simulink model "Two_Channel_PP_Teleoperation_kalman"  (R2022b)
settings: Solver=VariableStepAuto  StartTime=0.0  StopTime=10  RelTol=1e-9
values from neighbouring files (symbols this model uses):
  Amp = 15    [parameters.m]    (also in parameters_kalman.m)
  Be = 100    [parameters.m]    (also in parameters_kalman.m)
  Bh = 1    [parameters.m]    (also in parameters_kalman.m)
  Bm = 20*0.8    (= 16)    [parameters.m]    (also in parameters_kalman.m = 80)
  Bs = 4*Bm    (= 64)    [parameters.m]    (also in parameters_kalman.m = 300)
  delay = 10    [parameters.m]    (also in parameters_kalman.m)
  Dh = 20*0.8    (= 16)    [parameters.m]    (also in parameters_kalman.m)
  Dm = 1.3    [parameters.m]    (also in parameters_kalman.m)
  Ds = 1.2    [parameters.m]    (also in parameters_kalman.m)
  Fc = 1    [parameters.m]    (also in parameters_kalman.m)
  Flp = 5    [parameters.m]    (also in parameters_kalman.m)
  Jh = 1    [parameters.m]    (also in parameters_kalman.m)
  Ke = 200    [parameters.m]    (also in parameters_kalman.m)
  Km = 10*1    (= 10)    [parameters.m]    (also in parameters_kalman.m = 30)
  Ks = 4*Km    (= 40)    [parameters.m]    (also in parameters_kalman.m = 240)
  lambda = 150    [parameters_kalman.m]
  Mm = 0.5    [parameters.m]    (also in parameters_kalman.m)
  Ms = 2    [parameters.m]    (also in parameters_kalman.m)
  Ph = 10*1    (= 10)    [parameters.m]    (also in parameters_kalman.m)
  Ts = 0.001    [parameters.m]    (also in parameters_kalman.m)
  variance = 0.000001    (= 1e-06)    [parameters_kalman.m]
  xe = 1000    [parameters.m]    (also in parameters_kalman.m = 30)
undefined symbols (not defined in the file or in its folder): DiscIntNeverNeededParam
libraries: simulink x2
settings Model: Creator=uzair  LastModifiedBy=uzair

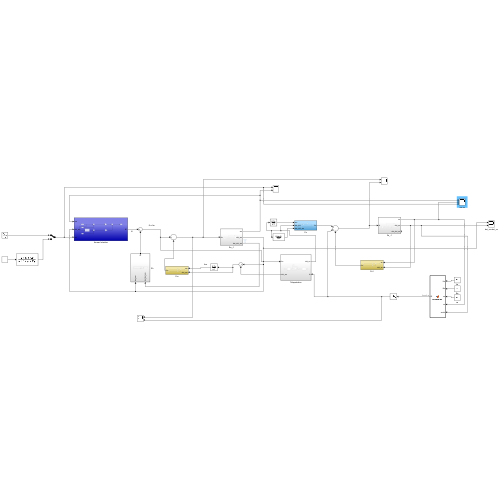
[thumbnail: Simulink's stored preview of the top-level diagram]
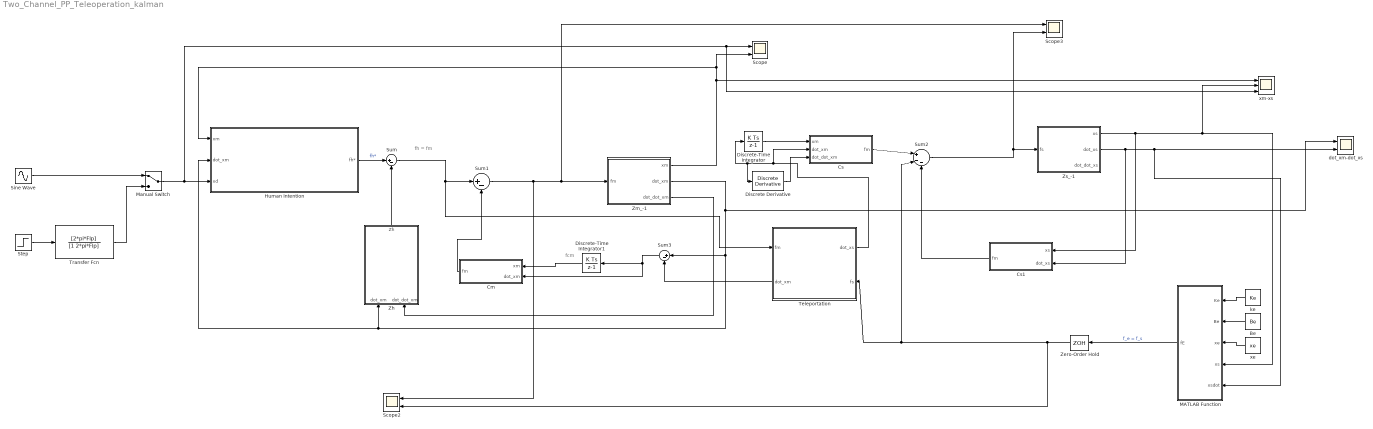
== system Two_Channel_PP_Teleoperation_kalman ==
  note: fcm
  note: fh = fm
  Be : Constant  Value=Be
  Cm : Subsystem
  Cs : Subsystem
  Cs1 : Subsystem
  Discrete Derivative : simulink/Discrete/Discrete Derivative  gainval=1.0  ICPrevScaledInput=0.0  OutMin=[]  OutMax=[]  OutDataType=fixdt(1, 16)  OutScaling=2^-10  DoSatur=off
  Discrete-Time Integrator : DiscreteIntegrator  SampleTime=Ts  ICPrevOutput=DiscIntNeverNeededParam  ICPrevScaledInput=DiscIntNeverNeededParam
  Discrete-Time Integrator1 : DiscreteIntegrator  SampleTime=Ts  ICPrevOutput=DiscIntNeverNeededParam  ICPrevScaledInput=DiscIntNeverNeededParam
  Human Intention : Subsystem
  MATLAB Function : MATLAB Function  TreatAsAtomicUnit=on
  Manual Switch : ManualSwitch
  Scope : Scope  NumInputPorts=2
  Scope2 : Scope  NumInputPorts=2
  Scope3 : Scope  NumInputPorts=2
  Sine Wave : Sin  Amplitude=Amp  Frequency=2*pi*Fc  SampleTime=0
  Step : Step  Time=0.5  After=Amp  SampleTime=0
  Sum : Sum  Inputs=|+-
  Sum1 : Sum  Inputs=|+-
  Sum2 : Sum  Inputs=|+--
  Sum3 : Sum  Inputs=|+-
  Teleportation : Subsystem
      settings: PortSchema="{\"entries\":[{\"content\":{\"sides\":[{\"content\":{\"connectorIds\":[\"In1\",\"Out2\"]},\"type\":\"ConnectorPlacement.EquallySpacedRectSide\",\"uuid\":\"b5f7abc7-c75d-4363-a17a-8f86c90608cd\"},{\"content\":{\"connectorIds\":[\"Out1\",\"In2\"],\"side\":\"RIGHT\"},\"type\":\"ConnectorPlacement.EquallySpacedRectSide\",\"uuid\":\"2ed87bee-e320-4c73-a1d3-1960a55b558d\"},{\"content\":{\"connectorIds\":[],\"side\":\"TOP\"},\"type\":\"ConnectorPlacement.EquallySpacedRectSide\",\"uuid\":\"65d6df07-20ed-40e6-978a-52c206d58fbe\"}]},\"type\":\"ConnectorPlacement.EquallySpacedConnector\",\"uuid\":\"b3d72d1f-cf16-401b-a692-293857f5cfdb\"}],\"packageUris\":[\"http://schema.mathworks.com/mf0/Connector/R2020b\"],\"version\":\"1.0\"}"
  Transfer Fcn : TransferFcn  Numerator=[2*pi*Flp]  Denominator=[1 2*pi*Flp]
  Zero-Order Hold : ZeroOrderHold  SampleTime=Ts
  Zh : Subsystem
  Zm_-1 : Subsystem
  Zs_-1 : Subsystem
  dot_xm-dot_xs : Scope  NumInputPorts=2
  ke : Constant  Value=Ke
  xe : Constant  Value=xe
  xm-xs : Scope  NumInputPorts=3
  wires:
  Sine Wave/1 -> Manual Switch/1
  Step/1 -> Transfer Fcn/1
  Transfer Fcn/1 -> Manual Switch/2
  Manual Switch/1 -> xm-xs/3, Scope/1, Human Intention/3(xd)
  Human Intention/1(fh*) -> Sum/1  "fh*"
  Zh/1(Zh) -> Sum/2
  Sum/1 -> Sum1/1, Teleportation/1(fm)
  Sum1/1 -> Scope2/1, Scope3/1, Zm_-1/1(fm)
  Zm_-1/3(dot_dot_xm) -> Zh/2(dot_dot_xm)
  Zm_-1/2(dot_xm) -> dot_xm-dot_xs/1, Human Intention/2(dot_xm), Zh/1(dot_xm), Sum3/1
  Cm/1(fm) -> Sum1/2
  Teleportation/2(dot_xm) -> Sum3/2
  Sum2/1 -> Scope3/2, Zs_-1/1(fs)
  xe/1 -> MATLAB Function/3(xe)
  Be/1 -> MATLAB Function/2(Be)
  ke/1 -> MATLAB Function/1(Ke)
  MATLAB Function/1(fE) -> Zero-Order Hold/1  "f_e = f_s"
  Zm_-1/1(xm) -> Scope/2, Human Intention/1(xm), xm-xs/1
  Cs/1(fm) -> Sum2/1
  Sum3/1 -> Cm/2(dot_xm), Discrete-Time Integrator1/1
  Discrete-Time Integrator1/1 -> Cm/1(xm)
  Zs_-1/2(dot_xs) -> Cs1/2(dot_xs), dot_xm-dot_xs/2, MATLAB Function/5(xsdot)
  Teleportation/1(dot_xs) -> Cs/2(dot_xm), Discrete Derivative/1, Discrete-Time Integrator/1
  Zs_-1/1(xs) -> Cs1/1(xs), xm-xs/2, MATLAB Function/4(xs)
  Zero-Order Hold/1 -> Teleportation/2(fs), Sum2/2, Scope2/2
  Discrete-Time Integrator/1 -> Cs/1(xm)
  Discrete Derivative/1 -> Cs/3(dot_dot_xm)
  Cs1/1(fm) -> Sum2/3

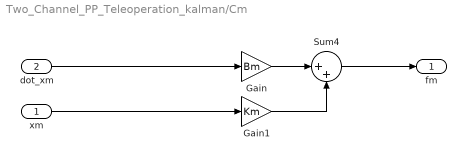
== system Two_Channel_PP_Teleoperation_kalman/Cm ==
  xm : Inport
  dot_xm : Inport  Port=2
  Gain : Gain  Gain=Bm
  Gain1 : Gain  Gain=Km
  Sum4 : Sum  Inputs=|++
  fm : Outport
  wires:
  Sum4/1 -> fm/1
  xm/1 -> Gain1/1
  Gain/1 -> Sum4/1
  Gain1/1 -> Sum4/2
  dot_xm/1 -> Gain/1

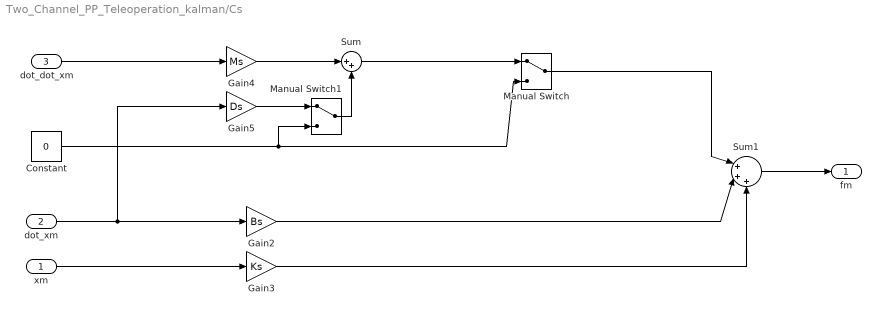
== system Two_Channel_PP_Teleoperation_kalman/Cs ==
  xm : Inport
  dot_xm : Inport  Port=2
  dot_dot_xm : Inport  Port=3
  Constant : Constant  Value=0
  Gain2 : Gain  Gain=Bs
  Gain3 : Gain  Gain=Ks
  Gain4 : Gain  Gain=Ms
  Gain5 : Gain  Gain=Ds
  Manual Switch : ManualSwitch
  Manual Switch1 : ManualSwitch
  Sum : Sum  Inputs=|++
  Sum1 : Sum  Inputs=|+++
  fm : Outport
  wires:
  Manual Switch1/1 -> Sum/2
  dot_xm/1 -> Gain5/1, Gain2/1
  Sum1/1 -> fm/1
  Sum/1 -> Manual Switch/1
  dot_dot_xm/1 -> Gain4/1
  Gain5/1 -> Manual Switch1/1
  Gain4/1 -> Sum/1
  xm/1 -> Gain3/1
  Gain2/1 -> Sum1/2
  Manual Switch/1 -> Sum1/1
  Gain3/1 -> Sum1/3
  Constant/1 -> Manual Switch1/2, Manual Switch/2

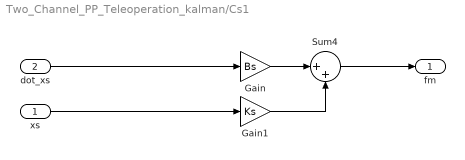
== system Two_Channel_PP_Teleoperation_kalman/Cs1 ==
  xs : Inport
  dot_xs : Inport  Port=2
  Gain : Gain  Gain=Bs
  Gain1 : Gain  Gain=Ks
  Sum4 : Sum  Inputs=|++
  fm : Outport
  wires:
  Sum4/1 -> fm/1
  xs/1 -> Gain1/1
  Gain/1 -> Sum4/1
  Gain1/1 -> Sum4/2
  dot_xs/1 -> Gain/1

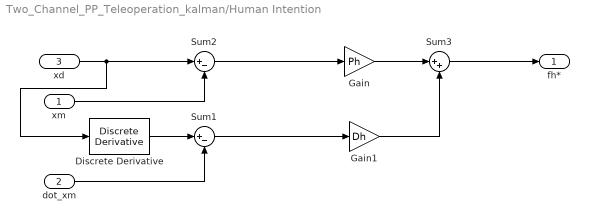
== system Two_Channel_PP_Teleoperation_kalman/Human Intention ==
  xm : Inport
  dot_xm : Inport  Port=2
  xd : Inport  Port=3
  Discrete Derivative : simulink/Discrete/Discrete Derivative  gainval=1.0  ICPrevScaledInput=0.0  OutMin=[]  OutMax=[]  OutDataType=fixdt(1, 16)  OutScaling=2^-10  DoSatur=off
  Gain : Gain  Gain=Ph
  Gain1 : Gain  Gain=Dh
  Sum1 : Sum  Inputs=|+-
  Sum2 : Sum  Inputs=|+-
  Sum3 : Sum  Inputs=|++
  fh* : Outport
  wires:
  xm/1 -> Sum2/2
  dot_xm/1 -> Sum1/2
  Sum2/1 -> Gain/1
  Sum1/1 -> Gain1/1
  Gain1/1 -> Sum3/2
  Gain/1 -> Sum3/1
  Sum3/1 -> fh*/1
  xd/1 -> Discrete Derivative/1, Sum2/1
  Discrete Derivative/1 -> Sum1/1

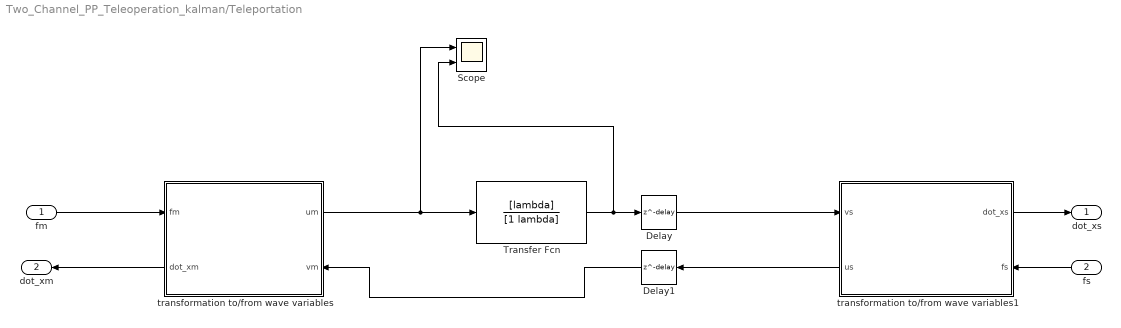
== system Two_Channel_PP_Teleoperation_kalman/Teleportation ==
  fm : Inport
  fs : Inport  Port=2
  Delay : Delay  DelayLength=delay  SampleTime=Ts
  Delay1 : Delay  DelayLength=delay  SampleTime=Ts
  Scope : Scope  NumInputPorts=2
  Transfer Fcn : TransferFcn  Numerator=[lambda]  Denominator=[1 lambda]
  transformation to/from wave variables : Subsystem
      settings: PortSchema="{\"entries\":[{\"content\":{\"sides\":[{\"content\":{\"connectorIds\":[\"In1\",\"Out2\"]},\"type\":\"ConnectorPlacement.EquallySpacedRectSide\",\"uuid\":\"b5f7abc7-c75d-4363-a17a-8f86c90608cd\"},{\"content\":{\"connectorIds\":[\"Out1\",\"In2\"],\"side\":\"RIGHT\"},\"type\":\"ConnectorPlacement.EquallySpacedRectSide\",\"uuid\":\"2ed87bee-e320-4c73-a1d3-1960a55b558d\"},{\"content\":{\"connectorIds\":[],\"side\":\"TOP\"},\"type\":\"ConnectorPlacement.EquallySpacedRectSide\",\"uuid\":\"65d6df07-20ed-40e6-978a-52c206d58fbe\"}]},\"type\":\"ConnectorPlacement.EquallySpacedConnector\",\"uuid\":\"b3d72d1f-cf16-401b-a692-293857f5cfdb\"}],\"packageUris\":[\"http://schema.mathworks.com/mf0/Connector/R2020b\"],\"version\":\"1.0\"}"
  transformation to/from wave variables1 : Subsystem
      settings: PortSchema="{\"entries\":[{\"content\":{\"sides\":[{\"content\":{\"connectorIds\":[\"In1\",\"Out2\"]},\"type\":\"ConnectorPlacement.EquallySpacedRectSide\",\"uuid\":\"b5f7abc7-c75d-4363-a17a-8f86c90608cd\"},{\"content\":{\"connectorIds\":[\"Out1\",\"In2\"],\"side\":\"RIGHT\"},\"type\":\"ConnectorPlacement.EquallySpacedRectSide\",\"uuid\":\"2ed87bee-e320-4c73-a1d3-1960a55b558d\"},{\"content\":{\"connectorIds\":[],\"side\":\"TOP\"},\"type\":\"ConnectorPlacement.EquallySpacedRectSide\",\"uuid\":\"65d6df07-20ed-40e6-978a-52c206d58fbe\"}]},\"type\":\"ConnectorPlacement.EquallySpacedConnector\",\"uuid\":\"b3d72d1f-cf16-401b-a692-293857f5cfdb\"}],\"packageUris\":[\"http://schema.mathworks.com/mf0/Connector/R2020b\"],\"version\":\"1.0\"}"
  dot_xs : Outport
  dot_xm : Outport  Port=2
  wires:
  fm/1 -> transformation to/from wave variables/1(fm)
  transformation to/from wave variables/2(dot_xm) -> dot_xm/1
  fs/1 -> transformation to/from wave variables1/2(fs)
  transformation to/from wave variables1/1(dot_xs) -> dot_xs/1
  transformation to/from wave variables1/2(us) -> Delay1/1
  Delay/1 -> transformation to/from wave variables1/1(vs)
  transformation to/from wave variables/1(um) -> Transfer Fcn/1, Scope/1
  Transfer Fcn/1 -> Scope/2, Delay/1
  Delay1/1 -> transformation to/from wave variables/2(vm)

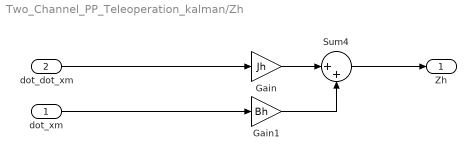
== system Two_Channel_PP_Teleoperation_kalman/Zh ==
  dot_xm : Inport
  dot_dot_xm : Inport  Port=2
  Gain : Gain  Gain=Jh
  Gain1 : Gain  Gain=Bh
  Sum4 : Sum  Inputs=|++
  Zh : Outport
  wires:
  dot_dot_xm/1 -> Gain/1
  Gain1/1 -> Sum4/2
  Gain/1 -> Sum4/1
  Sum4/1 -> Zh/1
  dot_xm/1 -> Gain1/1

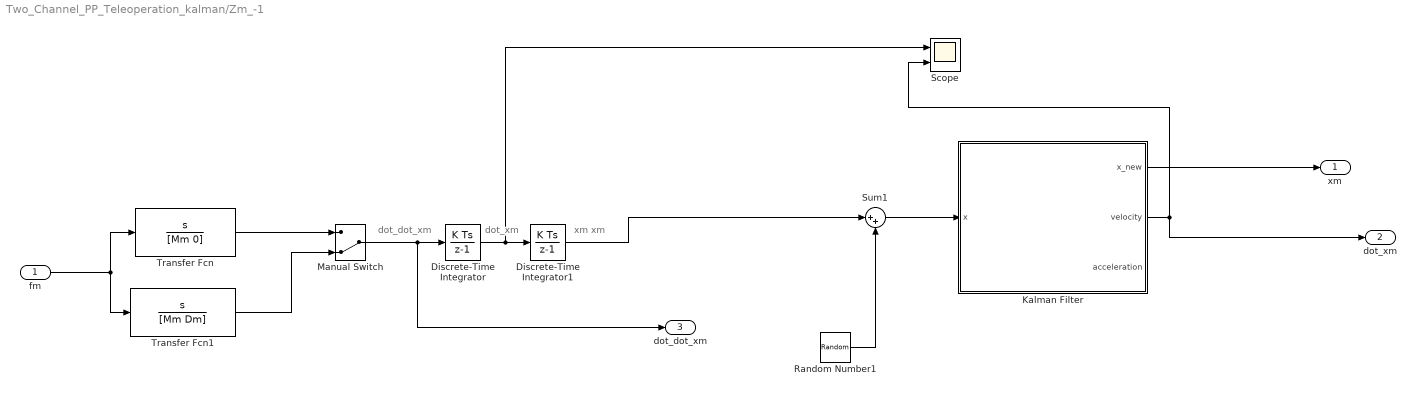
== system Two_Channel_PP_Teleoperation_kalman/Zm_-1 ==
  note: dot_dot_xm
  note: dot_xm
  note: xm
      | xm
  fm : Inport
  Discrete-Time Integrator : DiscreteIntegrator  SampleTime=Ts  ICPrevOutput=DiscIntNeverNeededParam  ICPrevScaledInput=DiscIntNeverNeededParam
  Discrete-Time Integrator1 : DiscreteIntegrator  SampleTime=Ts  ICPrevOutput=DiscIntNeverNeededParam  ICPrevScaledInput=DiscIntNeverNeededParam
  Kalman Filter : MATLAB Function  TreatAsAtomicUnit=on
  Manual Switch : ManualSwitch  CurrentSetting=0
  Random Number1 : RandomNumber  Variance=variance  SampleTime=Ts
  Scope : Scope  NumInputPorts=2
  Sum1 : Sum  Inputs=|++
  Transfer Fcn : TransferFcn  Numerator=[1 0]  Denominator=[Mm 0]
  Transfer Fcn1 : TransferFcn  Numerator=[1 0]  Denominator=[Mm Dm]
  xm : Outport
  dot_xm : Outport  Port=2
  dot_dot_xm : Outport  Port=3
  wires:
  Manual Switch/1 -> Discrete-Time Integrator/1, dot_dot_xm/1
  Discrete-Time Integrator1/1 -> Sum1/1
  Discrete-Time Integrator/1 -> Scope/1, Discrete-Time Integrator1/1
  fm/1 -> Transfer Fcn/1, Transfer Fcn1/1
  Transfer Fcn/1 -> Manual Switch/1
  Transfer Fcn1/1 -> Manual Switch/2
  Sum1/1 -> Kalman Filter/1(x)
  Random Number1/1 -> Sum1/2
  Kalman Filter/2(velocity) -> Scope/2, dot_xm/1
  Kalman Filter/1(x_new) -> xm/1

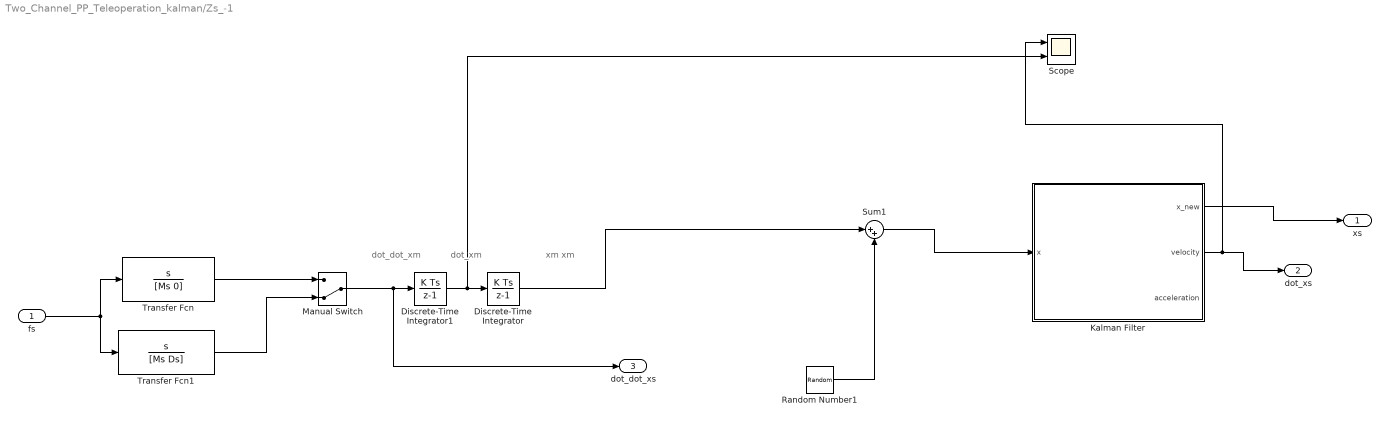
== system Two_Channel_PP_Teleoperation_kalman/Zs_-1 ==
  note: dot_dot_xm
  note: dot_xm
  note: xm
      | xm
  fs : Inport
  Discrete-Time Integrator : DiscreteIntegrator  SampleTime=Ts  ICPrevOutput=DiscIntNeverNeededParam  ICPrevScaledInput=DiscIntNeverNeededParam
  Discrete-Time Integrator1 : DiscreteIntegrator  SampleTime=Ts  ICPrevOutput=DiscIntNeverNeededParam  ICPrevScaledInput=DiscIntNeverNeededParam
  Kalman Filter : MATLAB Function  TreatAsAtomicUnit=on
  Manual Switch : ManualSwitch  CurrentSetting=0
  Random Number1 : RandomNumber  Variance=variance  SampleTime=Ts
  Scope : Scope  NumInputPorts=2
  Sum1 : Sum  Inputs=|++
  Transfer Fcn : TransferFcn  Numerator=[1 0]  Denominator=[Ms 0]
  Transfer Fcn1 : TransferFcn  Numerator=[1 0]  Denominator=[Ms Ds]
  xs : Outport
  dot_xs : Outport  Port=2
  dot_dot_xs : Outport  Port=3
  wires:
  Manual Switch/1 -> Discrete-Time Integrator1/1, dot_dot_xs/1
  Discrete-Time Integrator/1 -> Sum1/1
  fs/1 -> Transfer Fcn/1, Transfer Fcn1/1
  Transfer Fcn/1 -> Manual Switch/1
  Transfer Fcn1/1 -> Manual Switch/2
  Sum1/1 -> Kalman Filter/1(x)
  Random Number1/1 -> Sum1/2
  Kalman Filter/1(x_new) -> xs/1
  Kalman Filter/2(velocity) -> Scope/1, dot_xs/1
  Discrete-Time Integrator1/1 -> Scope/2, Discrete-Time Integrator/1

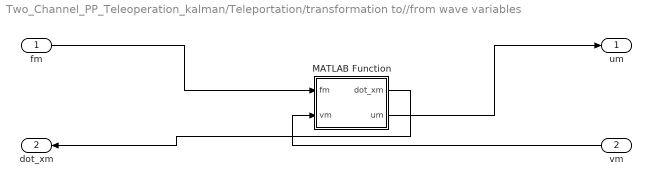
== system Two_Channel_PP_Teleoperation_kalman/Teleportation/transformation to//from wave variables ==
  fm : Inport
  vm : Inport  Port=2
  MATLAB Function : MATLAB Function  TreatAsAtomicUnit=on
  um : Outport
  dot_xm : Outport  Port=2
  wires:
  fm/1 -> MATLAB Function/1(fm)
  MATLAB Function/1(dot_xm) -> dot_xm/1
  MATLAB Function/2(um) -> um/1
  vm/1 -> MATLAB Function/2(vm)

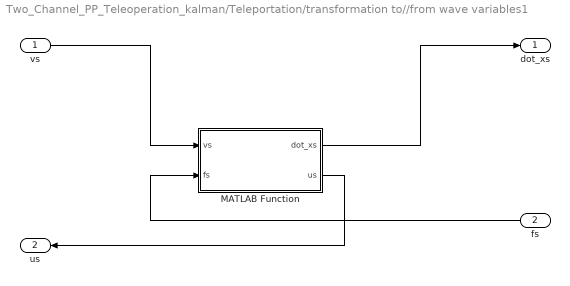
== system Two_Channel_PP_Teleoperation_kalman/Teleportation/transformation to//from wave variables1 ==
  vs : Inport
  fs : Inport  Port=2
  MATLAB Function : MATLAB Function  TreatAsAtomicUnit=on
  dot_xs : Outport
  us : Outport  Port=2
  wires:
  vs/1 -> MATLAB Function/1(vs)
  MATLAB Function/2(us) -> us/1
  MATLAB Function/1(dot_xs) -> dot_xs/1
  fs/1 -> MATLAB Function/2(fs)

== matlab function Two_Channel_PP_Teleoperation_kalman/Teleportation/transformation to//from wave variables/MATLAB Function ==
  data: fm input; dot_xm output; vm input; um output; b parameter
function [dot_xm, um] = fcn(fm, vm,b)
    um = sqrt(2/b)*fm-vm;
    dot_xm = (1/b)*(fm - sqrt(2*b)*vm);

== matlab function Two_Channel_PP_Teleoperation_kalman/MATLAB Function ==
  data: Ke input; fE output; Be input; xe input; xs input; xsdot input
function fE = environment(Ke, Be, xe, xs, xsdot)
    if xs > xe
        fE = Ke * (xs - xe) + Be * xsdot; % Plot both contributions Ke and Be
    else
        fE = 0;
    end
end

== matlab function Two_Channel_PP_Teleoperation_kalman/Teleportation/transformation to//from wave variables1/MATLAB Function ==
  data: vs input; dot_xs output; fs input; us output; b parameter
function [dot_xs, us]    = fcn(vs,fs,b)
    us = sqrt(2/b)*fs - vs;
    dot_xs = -(1/b)*(fs - sqrt(2*b)*vs);

== matlab function Two_Channel_PP_Teleoperation_kalman/Zs_-1/Kalman Filter ==
  data: x input; x_new output; paramsKalman parameter; velocity output; acceleration output
function [x_new, velocity, acceleration] = Kalman(x, paramsKalman)
    persistent x_k_x P_k_km1;

    if(isempty(x_k_x))
       x_k_x = [x;0;0];
       P_k_km1 = paramsKalman.P*eye(3);

    end


    P_kp1_k = paramsKalman.A*P_k_km1*paramsKalman.A' - paramsKalman.A*P_k_km1*paramsKalman.C'*pinv(paramsKalman.C*P_k_km1*paramsKalman.C'+paramsKalman.R)*paramsKalman.C*P_k_km1*paramsKalman.A'+paramsKalman.Q;
    k_kp1 = P_kp1_k*paramsKalman.C'*pinv(paramsKalman.C*P_kp1_k*paramsKalman.C'+paramsKalman.R);
    X_Kp1_kp1 = paramsKalman.A *x_k_x + k_kp1*(x - paramsKalman.C*paramsKalman.A*x_k_x);

    x_k_x = X_Kp1_kp1;
    P_k_km1 = P_kp1_k;

    x_new = X_Kp1_kp1(1);
    velocity = X_Kp1_kp1(2);
    acceleration = X_Kp1_kp1(3);

   
end

== matlab function Two_Channel_PP_Teleoperation_kalman/Zm_-1/Kalman Filter ==
  data: x input; x_new output; paramsKalman parameter; velocity output; acceleration output
function [x_new, velocity, acceleration] = Kalman(x, paramsKalman)
    persistent x_k_x P_k_km1;

    if(isempty(x_k_x))
       x_k_x = [x;0;0];
       P_k_km1 = paramsKalman.P*eye(3);

    end


    P_kp1_k = paramsKalman.A*P_k_km1*paramsKalman.A' - paramsKalman.A*P_k_km1*paramsKalman.C'*pinv(paramsKalman.C*P_k_km1*paramsKalman.C'+paramsKalman.R)*paramsKalman.C*P_k_km1*paramsKalman.A'+paramsKalman.Q;
    k_kp1 = P_kp1_k*paramsKalman.C'*pinv(paramsKalman.C*P_kp1_k*paramsKalman.C'+paramsKalman.R);
    X_Kp1_kp1 = paramsKalman.A *x_k_x + k_kp1*(x - paramsKalman.C*paramsKalman.A*x_k_x);

    x_k_x = X_Kp1_kp1;
    P_k_km1 = P_kp1_k;

    x_new = X_Kp1_kp1(1);
    velocity = X_Kp1_kp1(2);
    acceleration = X_Kp1_kp1(3);

   
end
